simulink model "zbiorniki_comp"  (R2024b)
settings: Solver=ode45  StartTime=0.0  StopTime=200  MaxStep=0.05  RelTol=1e-3
libraries: simulink x2
settings Model: Creator=gm54508  LastModifiedBy=gm54508

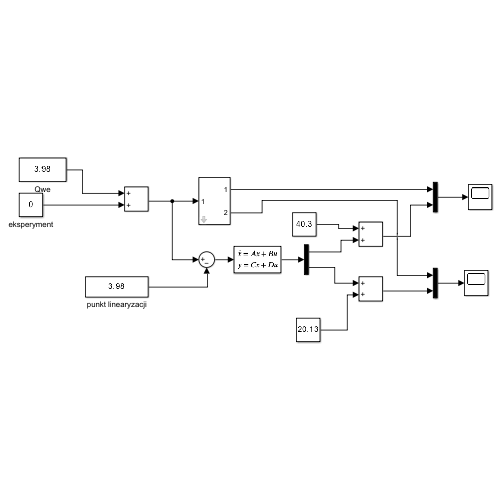
[thumbnail: Simulink's stored preview of the top-level diagram]
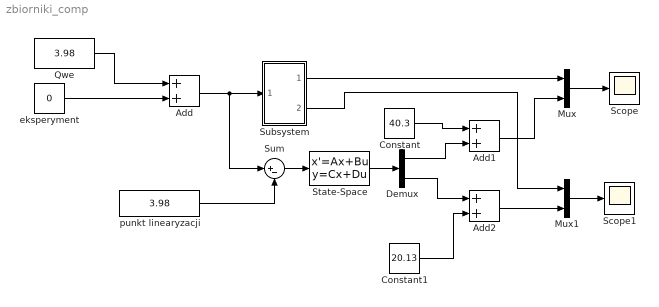
== system zbiorniki_comp ==
  Add : Sum
  Add1 : Sum
  Add2 : Sum
  Constant : Constant  Value=40.3
  Constant1 : Constant  Value=20.13
  Demux : Demux  Outputs=2
  Mux : Mux  Inputs=2
  Mux1 : Mux  Inputs=2
  Qwe : Constant  Value=3.98
  Scope : Scope
  Scope1 : Scope
  State-Space : StateSpace  A=[-0.098627165623799,0.098627165623799;0.049313582811899,-0.098676136422710]  B=[1;0]  C=[1,0;0,1]  D=[0;0]  InitialCondition=[4 - 40.03, 2 - 20]
  Subsystem : Subsystem  mask{h1=4, h2=2, s1=1, s2=2, swy1=0.2, swy2=0.2, fi1=1, fi2=1, g=9.81, qwe=3.98}
  Sum : Sum  Inputs=|+-
  eksperyment : Constant  Value=0
  punkt linearyzacji : Constant  Value=3.98
  wires:
  Add/1 -> Sum/1, Subsystem/1(In1)
  Subsystem/1(Out1) -> Mux/1
  Subsystem/2(Out2) -> Mux1/1
  eksperyment/1 -> Add/2
  Qwe/1 -> Add/1
  punkt linearyzacji/1 -> Sum/2
  Sum/1 -> State-Space/1
  State-Space/1 -> Demux/1
  Demux/1 -> Add1/2
  Constant/1 -> Add1/1
  Demux/2 -> Add2/1
  Constant1/1 -> Add2/2
  Add1/1 -> Mux/2
  Add2/1 -> Mux1/2
  Mux/1 -> Scope/1
  Mux1/1 -> Scope1/1

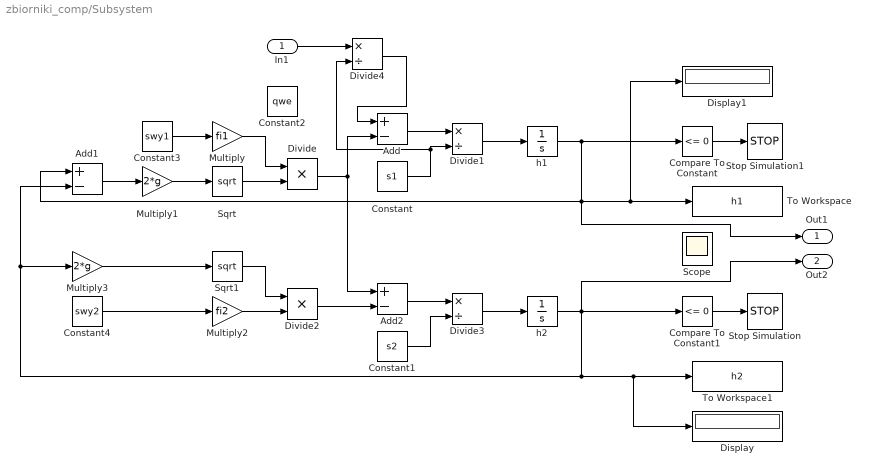
== system zbiorniki_comp/Subsystem ==
  In1 : Inport
  Add : Sum  Inputs=+-
  Add1 : Sum  Inputs=+-
  Add2 : Sum  Inputs=+-
  Compare To Constant : simulink/Logic and Bit Operations/Compare To Constant  relop=<=  const=0  OutDataTypeStr=boolean
  Compare To Constant1 : simulink/Logic and Bit Operations/Compare To Constant  relop=<=  const=0  OutDataTypeStr=boolean
  Constant : Constant  Value=s1
  Constant1 : Constant  Value=s2
  Constant2 : Constant  Value=qwe
  Constant3 : Constant  Value=swy1
  Constant4 : Constant  Value=swy2
  Display : Display
  Display1 : Display
  Divide : Product  Inputs=**
  Divide1 : Product  Inputs=*/
  Divide2 : Product  Inputs=**
  Divide3 : Product  Inputs=*/
  Divide4 : Product  Inputs=*/
  Multiply : Gain  Gain=fi1
  Multiply1 : Gain  Gain=2*g
  Multiply2 : Gain  Gain=fi2
  Multiply3 : Gain  Gain=2*g
  Scope : Scope  NumInputPorts=2
  Sqrt : Sqrt
  Sqrt1 : Sqrt
  Stop Simulation : Stop
  Stop Simulation1 : Stop
  To Workspace : ToWorkspace  VariableName=h1  SampleTime=-1
  To Workspace1 : ToWorkspace  VariableName=h2  SampleTime=-1
  h1 : Integrator  InitialCondition=h1
  h2 : Integrator  InitialCondition=h2
  Out1 : Outport
  Out2 : Outport  Port=2
  wires:
  Add1/1 -> Multiply1/1
  h2/1 -> Out2/1, Compare To Constant1/1, Display/1, To Workspace1/1, Add1/2, Multiply3/1
  Sqrt/1 -> Divide/2
  h1/1 -> Out1/1, Add1/1, Display1/1, To Workspace/1, Compare To Constant/1
  Divide2/1 -> Add2/2
  Constant4/1 -> Multiply2/1
  Constant3/1 -> Multiply/1
  Divide1/1 -> h1/1
  Multiply1/1 -> Sqrt/1
  Multiply2/1 -> Divide2/2
  Divide3/1 -> h2/1
  Multiply/1 -> Divide/1
  Sqrt1/1 -> Divide2/1
  Compare To Constant1/1 -> Stop Simulation/1
  Divide/1 -> Add2/1, Add/2
  Compare To Constant/1 -> Stop Simulation1/1
  Constant/1 -> Divide4/2, Divide1/2
  Constant1/1 -> Divide3/2
  Multiply3/1 -> Sqrt1/1
  Add/1 -> Divide1/1
  Add2/1 -> Divide3/1
  Divide4/1 -> Add/1
  In1/1 -> Divide4/1
